simulink model "lab2"  (R2021a)
settings: Solver=VariableStepAuto  StartTime=0.0  StopTime=10.0  RelTol=1e-3
undefined symbols (not defined in the file): K, N, sysol
libraries: cstblocks x2, simulink x1
settings Model: Creator=y.briere  LastModifiedBy=y.briere

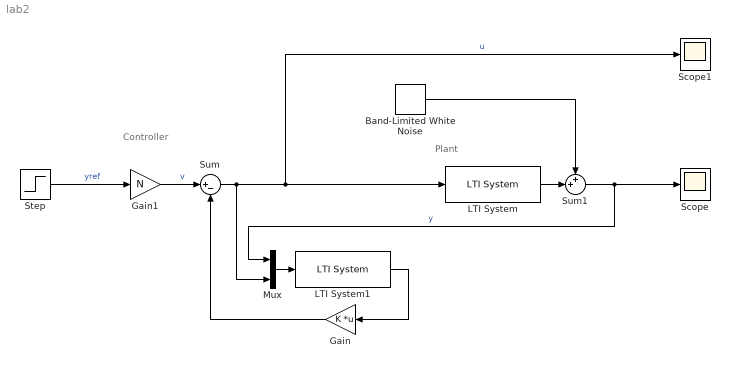
== system lab2 ==
  note: Plant
  note: Controller
  Band-Limited White Noise : simulink/Sources/Band-Limited White Noise  Cov=0.0000001  Ts=0.001  seed=[23341]
  Gain : Gain  Gain=K  Multiplication=Matrix(K*u)
  Gain1 : Gain  Gain=N
  LTI System : cstblocks/LTI System  sys=sysol(1,1)  IC=[]
  LTI System1 : cstblocks/LTI System  sys=sysobs  IC=[]
  Mux : Mux  Inputs=2
  Scope : Scope
  Scope1 : Scope
  Step : Step  SampleTime=0
  Sum : Sum  Inputs=|+-
  Sum1 : Sum  Inputs=++|
  wires:
  Mux/1 -> LTI System1/1
  Step/1 -> Gain1/1  "yref"
  Gain/1 -> Sum/2
  Gain1/1 -> Sum/1  "v"
  Sum/1 -> Scope1/1, LTI System/1, Mux/2  "u"
  LTI System1/1 -> Gain/1
  LTI System/1 -> Sum1/2
  Sum1/1 -> Mux/1, Scope/1  "y"
  Band-Limited White Noise/1 -> Sum1/1
